simulink model "TRN_KAISIM"  (R2022a)
settings: Solver=FixedStepAuto  StartTime=0.0  StopTime=300  FixedStep=0.04  RelTol=1e-3
PreLoadFcn:
  | load('BusStructureTRNsensor.mat');
  | load('BusStructureTRN.mat');
InitFcn:
  | load('BusStructureTRNsensor.mat');
  | load('BusStructureTRN.mat');
undefined symbols (not defined in the file or in its folder): Altitude_INS, Latitude_INS, Longitude_INS, residual, Result_Prev, TimeTag_Prev, TRN, TRNlib
libraries: simulink_extras x18, sharedtransform x3
(part 1 of 4)
settings Model: Creator=HSU  LastModifiedBy=ASCL
settings OptimizationCC: DefaultParameterBehavior=Inlined  UseDivisionForNetSlopeComputation=on  GainParamInheritBuiltInType=on  UseFloatMulNetSlope=on  PassReuseOutputArgsAs=Individual arguments  ZeroExternalMemoryAtStartup=off  ZeroInternalMemoryAtStartup=off  LifeSpan=Inf  OptimizeBlockOrder=speed  DifferentSizesBufferReuse=on  EfficientTunableParamExpr=on
settings DebuggingCC: ParameterTunabilityLossMsg=error  UnconnectedInputMsg=warning  UnconnectedOutputMsg=warning  UnconnectedLineMsg=warning  SFUnexpectedBacktrackingDiag=warning  SFNoUnconditionalDefaultTransitionDiag=warning
settings HardwareCC: ProdBitPerPointer=32  ProdBitPerSizeT=32  ProdBitPerPtrDiffT=32  ProdLargestAtomicInteger=Long  ProdLargestAtomicFloat=Double  ProdEndianess=BigEndian  ProdWordSize=32  ProdLongLongMode=on  ProdHWDeviceType=Freescale->MPC83xx
settings ModelReferenceCC: ModelReferenceNumInstancesAllowed=Single
settings SFSimCC: SimCustomHeaderCode="#include \"MAP.h\""  SimUserSources=MAP.c  SimUserLibraries=WS2_32.LIB  MATLABDynamicMemAlloc=off
settings RTWCC: SystemTargetFile=ert.tlc  GenCodeOnly=on  TemplateMakefile=ert_default_tmf  GenerateReport=on  RTWUseSimCustomCode=on  CustomHeaderCode="#include \"MAP.h\""  CustomSource=MAP.c  CustomLibrary=WS2_32.LIB  BuildConfiguration=Faster Runs  LaunchReport=on  GenerateCodeMetricsReport=on  DLArmComputeVersion=19.05
settings CodeAppCC: ForceParamTrailComments=on  IgnoreCustomStorageClasses=off  OperatorAnnotations=on  SimulinkDataObjDesc=on  SFDataObjDesc=on  MATLABFcnDesc=on  InsertBlockDesc=on  StateflowObjectComments=on  MATLABSourceComments=on  EnableCustomComments=on  ReqsInCode=on
settings ERTTargetCC: TargetLangStandard=C99 (ISO)  UtilityFuncGeneration=Shared location  GenerateSampleERTMain=on  SuppressErrorStatus=on  SupportAbsoluteTime=off  SupportNonFinite=off  SupportComplex=off  SupportVariableSizeSignals=on  ParenthesesLevel=Standards  CastingMode=Standards  InlinedParameterPlacement=NonHierarchical  ERTCustomFileTemplate=example_file_process.tlc  PreserveIfCondition=on  ConvertIfToSwitch=off  EnableSignedLeftShifts=off  EnableSignedRightShifts=off

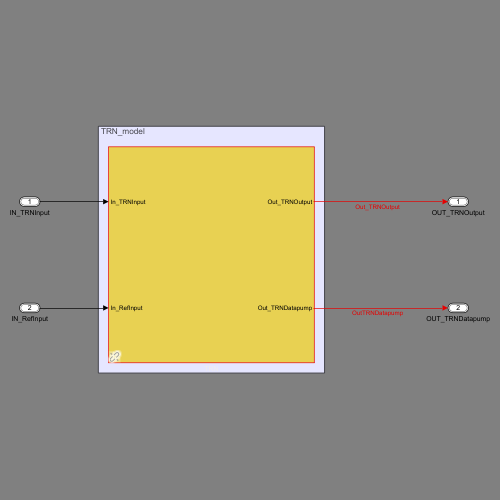
[thumbnail: Simulink's stored preview of the top-level diagram]
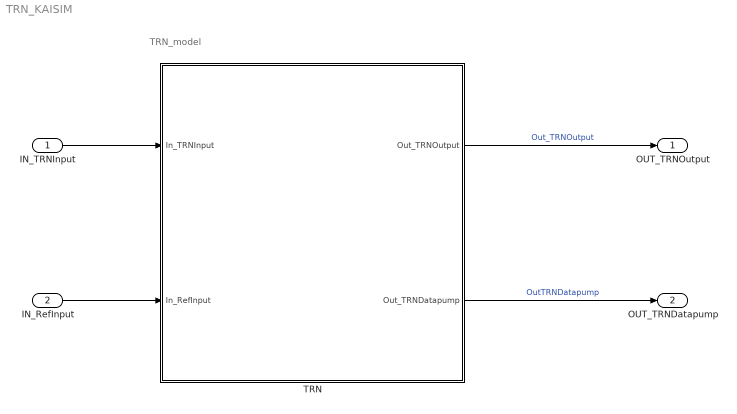
== system TRN_KAISIM ==
  note: TRN_model
  IN_TRNInput : Inport  OutDataTypeStr=Bus: TRNInput  Interpolate=off  BusOutputAsStruct=on
  IN_RefInput : Inport  Port=2  OutDataTypeStr=Bus: TRN_Ref  Interpolate=off  BusOutputAsStruct=on
  TRN : Subsystem  AncestorBlock=TRNlib/TRN
  OUT_TRNOutput : Outport  OutDataTypeStr=Bus: TRNOutput  BusOutputAsStruct=on
  OUT_TRNDatapump : Outport  Port=2  OutDataTypeStr=Bus: TRNDatapump  BusOutputAsStruct=on
  wires:
  IN_RefInput/1 -> TRN/2(In_RefInput)
  TRN/2(Out_TRNDatapump) -> OUT_TRNDatapump/1  "OutTRNDatapump"
  IN_TRNInput/1 -> TRN/1(In_TRNInput)
  TRN/1(Out_TRNOutput) -> OUT_TRNOutput/1  "Out_TRNOutput"

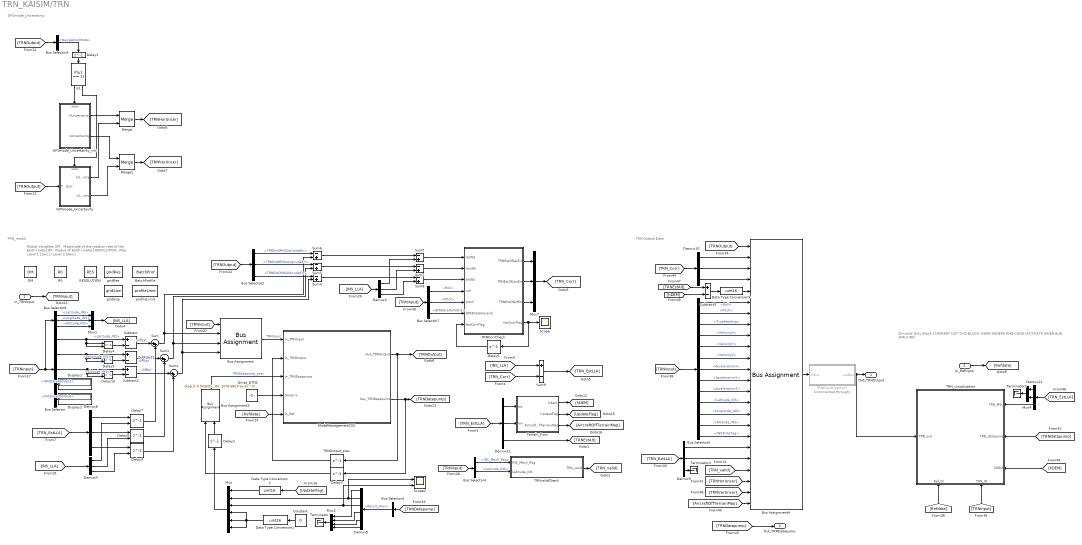
== system TRN_KAISIM/TRN ==
  note: GPSmode_Uncertainty
  note: Global Variables
      | OM : Magnitude of the rotation rate of the Earth [rad/s]
      | R0 : Radius of Earth [meter]
      | RESOLUTION : Map Level 1 [1arc] / Level 2 [3arc]
  note: TRN_modul
  note: TRN Output Data
  note: Simulink Only Block
      | COMMENT OUT THIS BLOCK WHEN GENERATING CODE
      | (ACTIVATE WHEN RUN SIMULINK)
  In_TRNInput : Inport  OutDataTypeStr=Bus: TRNInput
  In_RefInput : Inport  Port=2  OutDataTypeStr=Bus: TRN_Ref
  BatchProfile : DataStoreMemory  DataStoreName=BatchProf  ReadBeforeWriteMsg=warning  WriteAfterWriteMsg=warning  WriteAfterReadMsg=warning  ShowAdditionalParam=off  OutDataTypeStr=double  Dimensions=84200
  Bus Assignment : BusAssignment  AssignedSignals=Latitude_INS,Longitude_INS,Altitude_INS
  Bus Assignment3 : BusAssignment  AssignedSignals=Result_Prev
  Bus Assignment4 : BusAssignment  AssignedSignals=TRNEstOfINSLatitudeErr,TRNEstOfINSLongitudeErr,TRNEstOfINSAltitudeErr,TRNEstHeightAGL,TRN_Roll,TRN_Pitch,TRN_Yaw,TRN_VelocityX,TRN_VelocityY,TRN_VelocityZ,TRN_AccelerationX,TRN_AccelerationY,TRN_AccelerationZ,Latitude_INS,Longitude_INS,Altitude_INS,TRNTimeTag,TRNEstOfLatitude,TRNEstOfLongitude,TRN_valid,TRNHorUncertainty,TRNVerticalUncertainty,AircraftOffTerrainMap
  Bus Selector : BusSelector  OutputSignals=Latitude_INS,Longitude_INS,Altitude_INS,GPSDataNotValid,INSDataNotValid
  Bus Selector2 : BusSelector  OutputSignals=TRNEstOfINSLatitudeErr,TRNEstOfINSLongitudeErr,TRNEstOfINSAltitudeErr
  Bus Selector3 : BusSelector  OutputSignals=Result_Prev
  Bus Selector4 : BusSelector  OutputSignals=INS_Mech_flag,Latitude_INS
  Bus Selector5 : BusSelector  OutputSignals=Roll,Pitch,TrueHeading,VelocityX,VelocityY,VelocityZ,AccelerationX,AccelerationY,AccelerationZ,Latitude_INS,Longitude_INS,Altitude_INS,INSTimeTag
  Bus Selector6 : BusSelector  OutputSignals=Latitude_INS,Longitude_INS,Altitude_INS
  Bus Selector7 : BusSelector  OutputSignals=Roll,Pitch,GPSDataNotValid
  Bus Selector9 : BusSelector  OutputSignals=NavigationMode
  Constant : Constant  Value=0
  Data Type Conversion1 : DataTypeConversion  OutDataTypeStr=uint16  SaturateOnIntegerOverflow=off  RndMeth=Floor
  Data Type Conversion2 : DataTypeConversion  OutDataTypeStr=uint16  SaturateOnIntegerOverflow=off  RndMeth=Floor
  Data Type Conversion3 : DataTypeConversion  OutDataTypeStr=uint16  RndMeth=Nearest  SaturateOnIntegerOverflow=off
  Delay1 : Delay  DelayLength=1  InitialCondition=1
  Delay10 : Delay  DelayLength=1  InitialConditionSource=Input port  InitialCondition=35.2*pi/180
      settings: InputPortMap=u0,p4
  Delay2 : Delay  DelayLength=1  InitialCondition=0
  Delay3 : Delay  DelayLength=1  InitialCondition=0
  Delay4 : Delay  DelayLength=1  InitialConditionSource=Input port  InitialCondition=35.2*pi/180
      settings: InputPortMap=u0,p4
  Delay5 : Delay  DelayLength=1  InitialConditionSource=Input port  InitialCondition=35.2*pi/180
      settings: InputPortMap=u0,p4
  Delay6 : Delay  DelayLength=1
  Delay7 : Delay  DelayLength=1  InitialConditionSource=Input port  InitialCondition=0
      settings: InputPortMap=u0,p4
  Delay8 : Delay  DelayLength=1  InitialConditionSource=Input port  InitialCondition=0
      settings: InputPortMap=u0,p4
  Delay9 : Delay  DelayLength=1  InitialConditionSource=Input port  InitialCondition=0
      settings: InputPortMap=u0,p4
  Demux{3..4,8..12} (7 alike) : Demux  Outputs=3
  Demux5 : Demux  Outputs=6
  Display1 : Display
  Display2 : Display
  GPSmode_Uncertainty : Subsystem  TreatAsAtomicUnit=on
  GPSmode_Uncertainty_init : Subsystem  TreatAsAtomicUnit=on
  If1 : If  IfExpression=u1 == 1
  Merge : Merge
  Merge1 : Merge
  ModeManagementCSU : Stateflow chart  TreatAsAtomicUnit=on
      settings: RTWSystemCode=Nonreusable function  RTWFcnNameOpts=Use subsystem name
  Mux : Mux  Inputs=6
  Mux1 : Mux  Inputs=3
  Mux2 : Mux
  Mux4 : Mux  Inputs=2
  Mux7 : Mux  Inputs=3
  OM : DataStoreMemory  DataStoreName=OM  ReadBeforeWriteMsg=warning  WriteAfterWriteMsg=warning  WriteAfterReadMsg=warning  InitialValue=7.27e-5  ShowAdditionalParam=off
  Qmat_DTNS : Constant  Value=diag(([-0.043633231299858 0.06302577854424 -0.431484176187487 784 -1078 686]*1e-6).^2)
  R0 : DataStoreMemory  DataStoreName=R0  ReadBeforeWriteMsg=warning  WriteAfterWriteMsg=warning  WriteAfterReadMsg=warning  InitialValue=6378000  ShowAdditionalParam=off
  RESOLUTION : DataStoreMemory  DataStoreName=RES  ReadBeforeWriteMsg=warning  WriteAfterWriteMsg=warning  WriteAfterReadMsg=warning  InitialValue=1 * 0.000277777777777777 * 0.0174532925199433  ShowAdditionalParam=off  OutDataTypeStr=double
  Scope : Scope
  Scope2 : Scope  NumInputPorts=2
  Subtract{,1..3} (4 alike) : Sum  Inputs=+-
  Sum : Sum  Inputs=|++
  Sum1 : Sum  Inputs=|++
  Sum2 : Sum  Inputs=|++
  Sum{3..8} (6 alike) : Sum  Inputs=-+
  Sum9 : Sum  Inputs=+-
  TRNCorrCheck : MATLAB Function  TreatAsAtomicUnit=on
      settings: RTWSystemCode=Nonreusable function  RTWFcnNameOpts=Use subsystem name
  TRNEventInjector1 : MATLAB Function  Commented=through  TreatAsAtomicUnit=on
  TRNOutput_prev : Delay  DelayLength=1  InitialCondition=struct('NavigationMode', false);
  TRN_visualization : Subsystem
      settings: PortSchema="{\"entries\":[{\"content\":{\"sides\":[{\"content\":{\"connectorIds\":[\"In1\",\"In2\",\"In3\"]},\"type\":\"ConnectorPlacement.EquallySpacedRectSide\",\"uuid\":\"9b00cbc4-ca0d-429d-9536-38963fe71bc1\"},{\"content\":{\"connectorIds\":[\"In6\"],\"side\":\"RIGHT\"},\"type\":\"ConnectorPlacement.EquallySpacedRectSide\",\"uuid\":\"1db309fb-4b82-499a-a8dc-4a1ba85275fb\"},{\"content\":{\"connectorIds\":[\"In4\",\"In5\"],\"side\":\"TOP\"},\"type\":\"ConnectorPlacement.EquallySpacedRectSide\",\"uuid\":\"7e2d2316-30f0-423f-b46b-636ee0f4a770\"}]},\"type\":\"ConnectorPlacement.EquallySpacedConnector\",\"uuid\":\"aa6e905d-ed4c-45ad-a850-3c33939aad22\"}],\"packageUris\":[\"http://schema.mathworks.com/mf0/Connector/R2020b\"],\"version\":\"1.0\"}"
  TRNvalidCheck : MATLAB Function  TreatAsAtomicUnit=on
      settings: RTWSystemCode=Nonreusable function  RTWFcnNameOpts=Use subsystem name
  Terminator : Terminator
  Terminator3 : Terminator
  Terminator4 : Terminator
  Terrain_Func : Subsystem
  gridRes : DataStoreMemory  DataStoreName=gridRes  ReadBeforeWriteMsg=warning  WriteAfterWriteMsg=warning  WriteAfterReadMsg=warning  InitialValue=0.3  ShowAdditionalParam=off  OutDataTypeStr=double
  gridSize : DataStoreMemory  DataStoreName=gridSize  ReadBeforeWriteMsg=warning  WriteAfterWriteMsg=warning  WriteAfterReadMsg=warning  InitialValue=20  ShowAdditionalParam=off  OutDataTypeStr=double
  profileLimit : DataStoreMemory  DataStoreName=profileLimit  ReadBeforeWriteMsg=warning  WriteAfterWriteMsg=warning  WriteAfterReadMsg=warning  InitialValue=20  ShowAdditionalParam=off  OutDataTypeStr=uint16
  Out_TRNOutput : Outport  OutDataTypeStr=Bus: TRNOutput  VectorParamsAs1DForOutWhenUnconnected=off
  Out_TRNDatapump : Outport  Port=2  OutDataTypeStr=Bus: TRNDatapump  VectorParamsAs1DForOutWhenUnconnected=off
  wires:
  If1/1 -> GPSmode_Uncertainty_init/Action
  If1/2 -> GPSmode_Uncertainty/Action
  GPSmode_Uncertainty_init/1(hUncertainty) -> Merge/1
  GPSmode_Uncertainty/1(hUncertainty) -> Merge/2
  GPSmode_Uncertainty_init/2(vUncertainty) -> Merge1/1
  GPSmode_Uncertainty/2(vUncertainty) -> Merge1/2
  Bus Selector9/1 -> Delay1/1  "<NavigationMode>"
  Merge/1 -> [TRNHorUncer]
  Merge1/1 -> [TRNVerUncer]
  [TRNOutput] -> Bus Selector9/1
  [TRNOutput] -> GPSmode_Uncertainty/1(TRNOutput)
  Delay1/1 -> If1/1
  Delay10/1 -> Subtract2/2
  [TRN_Corr] -> Sum9/2
  Mux/1 -> Delay2/1
  TRNCorrCheck/4(NotCorrFlag) -> Scope/1, Delay6/1
  Bus Selector/5 -> Display2/1  "<INSDataNotValid>"
  In_TRNInput/1 -> [TRNinput]
  Bus Selector/4 -> Display1/1  "<GPSDataNotValid>"
  Bus Selector6/1 -> Mux1/1  "<Latitude_INS>"
  [TRNOutput] -> Bus Selector2/1
  Bus Assignment3/1 -> ModeManagementCSU/3(In_TRNDatapump)  "TRNDatapump_prev"
  [INS_LLA] -> Demux4/1
  Demux4/3 -> Delay9/2
  Delay7/1 -> Sum/2
  Bus Selector7/3 -> TRNCorrCheck/6(GPSDataNotvalid)  "<GPSDataNotValid>"
  Demux4/2 -> Delay8/2
  Demux4/1 -> Delay7/2
  [TRNinput] -> Bus Selector7/1
  ModeManagementCSU/2(Out_TRNDatapump) -> Delay3/1, [TRNDatapump]
  Bus Selector7/1 -> TRNCorrCheck/4(roll)  "<Roll>"
  [TRNinput] -> Bus Selector6/1, Bus Selector/1
  [INS_LLA] -> Demux3/1
  Bus Selector6/2 -> Mux1/2  "<Longitude_INS>"
  Demux11/1 -> Terrain_Func/1(lat)
  Delay6/1 -> TRNCorrCheck/7("NotCorrFlag ")
  Sum9/1 -> [TRN_EstLLA]
  Bus Selector6/3 -> Mux1/3  "<Altitude_INS>"
  Mux7/1 -> [TRN_Corr]
  TRNCorrCheck/1(TRNEstOfLatErr) -> Mux7/1
  Subtract2/1 -> Sum2/1  "diffAlt"
  Delay9/1 -> Sum2/2
  [TRN_EstLLA] -> Demux8/1
  Demux8/3 -> Delay9/1
  Sum8/1 -> TRNCorrCheck/3(altINS)
  Sum7/1 -> TRNCorrCheck/2(lonINS)
  Sum/1 -> Sum6/2, Bus Assignment/2
  Bus Selector2/1 -> Sum6/1  "<TRNEstOfINSLatitudeErr>"
  Subtract/1 -> Sum/1  "diffLat"
  Delay8/1 -> Sum1/2
  Sum3/1 -> Sum7/1
  TRNOutput_prev/1 -> ModeManagementCSU/2(In_TRNOutput)
  Bus Selector/2 -> Subtract1/1, Delay5/2, Delay5/1  "<Longitude_INS>"
  Delay5/1 -> Subtract1/2
  Subtract1/1 -> Sum1/1  "diffLon"
  Bus Assignment/1 -> ModeManagementCSU/1(In_TRNInput)  "TRNInput"
  [INS_LLA] -> Sum9/1
  [TRNinput] -> Bus Assignment/1
  Terrain_Func/1(hdem) -> [hDEM]
  Delay4/1 -> Subtract/2
  Sum5/1 -> TRNCorrCheck/1(latINS)
  Demux3/1 -> Sum5/2
  Demux11/2 -> Terrain_Func/2(lon)
  Bus Selector2/2 -> Sum3/1  "<TRNEstOfINSLongitudeErr>"
  Demux3/3 -> Sum8/2
  Mux1/1 -> [INS_LLA]
  Demux3/2 -> Sum7/2
  Demux8/1 -> Delay7/1
  [TRN_EstLLA] -> Demux11/1
  [UpdateFlag] -> Data Type Conversion2/1
  Sum1/1 -> Sum3/2, Bus Assignment/3
  Terrain_Func/3(AircraftOffTerrainMap) -> [AircraftOffTerrainMap]
  Delay3/1 -> Bus Assignment3/1
  Demux11/3 -> [TRNEstAlt]
  Terrain_Func/2(Updateflag) -> [UpdateFlag]
  Constant/1 -> Data Type Conversion1/1
  TRNvalidCheck/1(TRN_valid) -> [TRN_valid]
  TRNCorrCheck/2(TRNEstOfLonErr) -> Mux7/2
  Demux8/2 -> Delay8/1
  Bus Selector/1 -> Delay4/2, Delay4/1, Subtract/1  "<Latitude_INS>"
  Bus Selector/3 -> Delay10/1, Delay10/2, Subtract2/1  "<Altitude_INS>"
  Delay2/1 -> Bus Assignment3/2
  TRNCorrCheck/3(TRNEstOfaltErr) -> Mux7/3
  Bus Selector2/3 -> Sum4/1  "<TRNEstOfINSAltitudeErr>"
  Bus Selector7/2 -> TRNCorrCheck/5(pitch)  "<Pitch>"
  ModeManagementCSU/1(Out_TRNOutput) -> [TRNOutput], TRNOutput_prev/1
  [TRNinput] -> Bus Selector4/1
  Data Type Conversion1/1 -> Mux/4, Mux/6, Mux/5
  Data Type Conversion2/1 -> Mux/1
  Sum2/1 -> Sum4/2, Bus Assignment/4
  Bus Selector4/1 -> TRNvalidCheck/1(INS_Mech_flag)  "<INS_Mech_flag>"
  Bus Selector4/2 -> TRNvalidCheck/2(Latitude_INS)  "<Latitude_INS>"
  Qmat_DTNS/1 -> ModeManagementCSU/4(Qmatrix)
  [Refdata] -> ModeManagementCSU/5(In_Ref)
  Bus Selector3/1 -> Demux5/1  "<Result_Prev>"
  [TRNDatapump] -> Bus Selector3/1
  Sum4/1 -> Sum8/1
  Sum6/1 -> Sum5/1
  Demux5/2 -> Mux/2, Scope2/1
  Demux5/3 -> Mux/3, Scope2/2
  Mux2/1 -> Terminator/1
  Demux5/1 -> Mux2/1
  Demux5/4 -> Mux2/2
  Demux5/5 -> Mux2/3
  Demux5/6 -> Mux2/4
  [TRNDatapump] -> Out_TRNDatapump/1
  Bus Selector5/8 -> Bus Assignment4/13  "<AccelerationY>"
  [TRNDatapump] -> TRN_visualization/2(TRN_datapump)
  Demux9/3 -> Terminator4/1
  [Refdata] -> TRN_visualization/5(Ref_IN)
  Bus Selector5/12 -> Bus Assignment4/17  "<Altitude_INS>"
  [TRN_EstLLA] -> Demux12/1
  Bus Selector5/3 -> Bus Assignment4/8  "<TrueHeading>"
  Demux9/2 -> Bus Assignment4/20
  [TRNVerUncer] -> Bus Assignment4/23
  [hDEM] -> Subtract3/2
  Bus Selector5/6 -> Bus Assignment4/11  "<VelocityZ>"
  [TRNOutput] -> Bus Assignment4/1
  Demux12/1 -> Mux4/1
  [TRN_EstLLA] -> Demux9/1
  Bus Selector5/2 -> Bus Assignment4/7  "<Pitch>"
  [hDEM] -> TRN_visualization/1(hDEM)
  [AircraftOffTerrainMap] -> Bus Assignment4/24
  Demux12/3 -> TRN_visualization/3(TRN_MSL)
  [TRN_Corr] -> Demux10/1
  Demux10/1 -> Bus Assignment4/2
  [TRNinput] -> TRN_visualization/4(TRN_IN)
  Bus Assignment4/1 -> TRNEventInjector1/1(inBus)
  Bus Selector5/1 -> Bus Assignment4/6  "<Roll>"
  Bus Selector5/4 -> Bus Assignment4/9  "<VelocityX>"
  Bus Selector5/13 -> Bus Assignment4/18  "<INSTimeTag>"
  Bus Selector5/5 -> Bus Assignment4/10  "<VelocityY>"
  Demux10/2 -> Bus Assignment4/3
  Bus Selector5/10 -> Bus Assignment4/15  "<Latitude_INS>"
  Data Type Conversion3/1 -> Bus Assignment4/5
  Bus Selector5/7 -> Bus Assignment4/12  "<AccelerationX>"
  In_RefInput/1 -> [Refdata]
  Demux9/1 -> Bus Assignment4/19
  Mux4/1 -> Terminator3/1
  Demux12/2 -> Mux4/2
  Bus Selector5/9 -> Bus Assignment4/14  "<AccelerationZ>"
  Demux10/3 -> Bus Assignment4/4
  Subtract3/1 -> Data Type Conversion3/1
  [TRNinput] -> Bus Selector5/1
  [TRN_valid] -> Bus Assignment4/21
  Bus Selector5/11 -> Bus Assignment4/16  "<Longitude_INS>"
  [TRNHorUncer] -> Bus Assignment4/22
  [TRNEstAlt] -> Subtract3/1
  TRNEventInjector1/1(outBus) -> TRN_visualization/6(TRN_out), Out_TRNOutput/1

== system TRN_KAISIM/TRN/GPSmode_Uncertainty ==
  TRNOutput : Inport
  Action Port : ActionPort  ActionPortLabel=else
  Bus Selector : BusSelector  OutputSignals=TRNHorUncertainty,TRNVerticalUncertainty
  Scope : Scope  NumInputPorts=2
  hUncertainty : Outport
  vUncertainty : Outport  Port=2
  wires:
  TRNOutput/1 -> Bus Selector/1
  Bus Selector/1 -> Scope/1, hUncertainty/1  "<TRNHorUncertainty>"
  Bus Selector/2 -> vUncertainty/1, Scope/2  "<TRNVerticalUncertainty>"

== system TRN_KAISIM/TRN/GPSmode_Uncertainty_init ==
  Action Port : ActionPort  ActionPortLabel=if(u1 == 1)
  Uncertainty_init : MATLAB Function  TreatAsAtomicUnit=on
  hUncertainty : Outport
  vUncertainty : Outport  Port=2
  wires:
  Uncertainty_init/1(hUncertainty) -> hUncertainty/1
  Uncertainty_init/2(vUncertainty) -> vUncertainty/1

== system TRN_KAISIM/TRN/ModeManagementCSU/AcquisitionCSU ==
  In_TRNInput : Inport  OutDataTypeStr=Bus: TRNInput  PortDimensions=1
  In_TRNDatapump : Inport  Port=2  OutDataTypeStr=Bus: TRNDatapump  PortDimensions=1
  f : TriggerPort  TriggerType=function-call  VariantControl=Variant
      settings: CopyFcn=Stateflow.SLINSF.SimulinkMan.removeBlockPreDeleteFcn  PreDeleteFcn=Stateflow.SLINSF.SimulinkMan.unsafePredeleteFcn
  AcquisitionCSU : Subsystem  TreatAsAtomicUnit=on
      settings: RTWSystemCode=Nonreusable function  RTWFcnNameOpts=Use subsystem name
  MAD : Outport  VectorParamsAs1DForOutWhenUnconnected=off
  profileCnt : Outport  Port=2  VectorParamsAs1DForOutWhenUnconnected=off
  posUpdate : Outport  Port=3  VectorParamsAs1DForOutWhenUnconnected=off
  residual : Outport  Port=4  VectorParamsAs1DForOutWhenUnconnected=off
  wires:
  In_TRNInput/1 -> AcquisitionCSU/1(In_TRNInput)
  In_TRNDatapump/1 -> AcquisitionCSU/2(In_TRNDatapump)
  AcquisitionCSU/1(MAD) -> MAD/1
  AcquisitionCSU/2(profileCnt) -> profileCnt/1
  AcquisitionCSU/3(posUpdate) -> posUpdate/1
  AcquisitionCSU/4(residual) -> residual/1

== system TRN_KAISIM/TRN/ModeManagementCSU/CorrelationValid ==
  In_TRNDatapump : Inport  OutDataTypeStr=Bus: TRNDatapump  PortDimensions=1
  In_TRNInput : Inport  Port=2  OutDataTypeStr=Bus: TRNInput  PortDimensions=1
  posUpdate : Inport  Port=3  OutDataTypeStr=double  PortDimensions=2
  In_Ref : Inport  Port=4  OutDataTypeStr=Bus: TRN_Ref  PortDimensions=1
  f : TriggerPort  TriggerType=function-call  VariantControl=Variant
      settings: CopyFcn=Stateflow.SLINSF.SimulinkMan.removeBlockPreDeleteFcn  PreDeleteFcn=Stateflow.SLINSF.SimulinkMan.unsafePredeleteFcn
  Bus Selector1 : BusSelector  OutputSignals=MAD,profileCnt
  Bus Selector2 : BusSelector  OutputSignals=GPSDataNotValid
  Bus Selector3 : BusSelector  OutputSignals=Latitude,Longitude
  CorrelationValid function : MATLAB Function  TreatAsAtomicUnit=on
  Terminator1 : Terminator
  Terminator4 : Terminator
  TRNEstLatErr : Outport  VectorParamsAs1DForOutWhenUnconnected=off
  TRNEstLonErr : Outport  Port=2  VectorParamsAs1DForOutWhenUnconnected=off
  TRNEstAltErr : Outport  Port=3
  profileCnt : Outport  Port=4  OutDataTypeStr=uint32
  NavigationMode : Outport  Port=5  OutDataTypeStr=boolean
  AircraftPositionCorrectionValid : Outport  Port=6
  wires:
  In_TRNDatapump/1 -> Bus Selector1/1
  Bus Selector1/2 -> CorrelationValid function/3("profileCnt ")  "<profileCnt>"
  Bus Selector2/1 -> CorrelationValid function/4(GPSDataNotValid)  "<GPSDataNotValid>"
  In_TRNInput/1 -> Bus Selector2/1
  Bus Selector1/1 -> CorrelationValid function/2(MAD)  "<MAD>"
  CorrelationValid function/1(TRNEstOfINSLatitudeErr) -> TRNEstLatErr/1
  CorrelationValid function/2(TRNEstOfINSLongitudeErr) -> TRNEstLonErr/1
  CorrelationValid function/3(TRNEstOfINSAltitudeErr) -> TRNEstAltErr/1
  CorrelationValid function/4(profileCnt) -> profileCnt/1
  CorrelationValid function/5(NavigationMode) -> NavigationMode/1
  CorrelationValid function/6(AircraftPositionCorrectionValid) -> AircraftPositionCorrectionValid/1
  posUpdate/1 -> CorrelationValid function/1(posUpdate)
  In_Ref/1 -> Bus Selector3/1
  Bus Selector3/1 -> Terminator4/1  "<Latitude>"
  Bus Selector3/2 -> Terminator1/1  "<Longitude>"

== system TRN_KAISIM/TRN/ModeManagementCSU/TrackingCSU ==
  In_TRNInput : Inport  OutDataTypeStr=Bus: TRNInput  PortDimensions=1
  Qmatrix : Inport  Port=2  OutDataTypeStr=double  PortDimensions=[6 6]
  In_TRNDatapump : Inport  Port=3  OutDataTypeStr=Bus: TRNDatapump  PortDimensions=1
  f : TriggerPort  TriggerType=function-call  VariantControl=Variant
      settings: CopyFcn=Stateflow.SLINSF.SimulinkMan.removeBlockPreDeleteFcn  PreDeleteFcn=Stateflow.SLINSF.SimulinkMan.unsafePredeleteFcn
  TrackingCSU_20230430 : Subsystem  TreatAsAtomicUnit=on
      settings: RTWSystemCode=Nonreusable function  RTWFcnNameOpts=Use subsystem name
  latINSErrTRN : Outport  VectorParamsAs1DForOutWhenUnconnected=off
  lonINSErrTRN : Outport  Port=2  VectorParamsAs1DForOutWhenUnconnected=off
  altINSErrTRN : Outport  Port=3  VectorParamsAs1DForOutWhenUnconnected=off
  hUncertainty : Outport  Port=4  VectorParamsAs1DForOutWhenUnconnected=off
  vUncertainty : Outport  Port=5  VectorParamsAs1DForOutWhenUnconnected=off
  Out_TRNDatapump : Outport  Port=6  VectorParamsAs1DForOutWhenUnconnected=off
  wires:
  In_TRNInput/1 -> [In_TRNinput]
  Qmatrix/1 -> [Qmat]
  In_TRNDatapump/1 -> [In_TRNDatapump]
  [In_TRNinput] -> TrackingCSU_20230430/1(In_TRNInput)
  [In_TRNDatapump] -> TrackingCSU_20230430/3(In_TRNDatapump)
  TrackingCSU_20230430/1(latINSErrTRN) -> latINSErrTRN/1
  TrackingCSU_20230430/2(lonINSErrTRN) -> lonINSErrTRN/1
  TrackingCSU_20230430/3(altINSErrTRN) -> altINSErrTRN/1
  TrackingCSU_20230430/5(vUncertainty) -> vUncertainty/1
  [Qmat] -> TrackingCSU_20230430/2(Qmatrix)
  TrackingCSU_20230430/4(hUncertainty) -> hUncertainty/1
  TrackingCSU_20230430/6(TRN_Datapump) -> Out_TRNDatapump/1

== system TRN_KAISIM/TRN/ModeManagementCSU/ValidityCheck ==
  continuousValid : Inport  OutDataTypeStr=boolean  PortDimensions=1
  latINSErrTRN : Inport  Port=2  OutDataTypeStr=double  PortDimensions=1
  lonINSErrTRN : Inport  Port=3  OutDataTypeStr=double  PortDimensions=1
  altINSErrTRN : Inport  Port=4  OutDataTypeStr=double  PortDimensions=1
  Result_prev : Inport  Port=5  OutDataTypeStr=uint16  PortDimensions=6
  f : TriggerPort  TriggerType=function-call  VariantControl=Variant
      settings: CopyFcn=Stateflow.SLINSF.SimulinkMan.removeBlockPreDeleteFcn  PreDeleteFcn=Stateflow.SLINSF.SimulinkMan.unsafePredeleteFcn
  Data Type Conversion : DataTypeConversion  OutDataTypeStr=boolean  SaturateOnIntegerOverflow=off  RndMeth=Floor
  Demux : Demux  Outputs=6
  Mux : Mux  Inputs=5
  Terminator : Terminator
  ValidityCheck : MATLAB Function  TreatAsAtomicUnit=on
      settings: RTWFcnNameOpts=Use subsystem name
  TRNEstOfINSLatitudeErr : Outport  VectorParamsAs1DForOutWhenUnconnected=off
  TRNEstOfINSLongitudeErr : Outport  Port=2
  TRNEstOfINSAltitudeErr : Outport  Port=3
  AircraftPositionCorrectionValid : Outport  Port=4  OutDataTypeStr=boolean
  wires:
  ValidityCheck/4(AircraftPositionCorrectionValid) -> AircraftPositionCorrectionValid/1
  continuousValid/1 -> ValidityCheck/1(continuousValid)
  latINSErrTRN/1 -> ValidityCheck/2(latINSErrTRN)
  lonINSErrTRN/1 -> ValidityCheck/3(lonINSErrTRN)
  altINSErrTRN/1 -> ValidityCheck/4(altINSErrTRN)
  ValidityCheck/3(TRNEstOfINSAltitudeErr) -> TRNEstOfINSAltitudeErr/1
  ValidityCheck/2(TRNEstOfINSLongitudeErr) -> TRNEstOfINSLongitudeErr/1
  ValidityCheck/1(TRNEstOfINSLatitudeErr) -> TRNEstOfINSLatitudeErr/1
  Result_prev/1 -> Demux/1
  Data Type Conversion/1 -> ValidityCheck/5(velFlag)
  Demux/3 -> Data Type Conversion/1
  Demux/1 -> Mux/1
  Demux/2 -> Mux/2
  Demux/4 -> Mux/3
  Demux/5 -> Mux/4
  Demux/6 -> Mux/5
  Mux/1 -> Terminator/1

== system TRN_KAISIM/TRN/ModeManagementCSU/Ver_FlightPath_Angle ==
  In_TRNInput : Inport  OutDataTypeStr=Bus: TRNInput  PortDimensions=1
  f : TriggerPort  TriggerType=function-call  VariantControl=Variant
      settings: CopyFcn=Stateflow.SLINSF.SimulinkMan.removeBlockPreDeleteFcn  PreDeleteFcn=Stateflow.SLINSF.SimulinkMan.unsafePredeleteFcn
  Bus Selector1 : BusSelector  OutputSignals=VelocityX,VelocityY,VelocityZ,Roll,Pitch,TrueHeading
  Degrees to Radians1 : simulink_extras/Transformations/Degrees to Radians
  Degrees to Radians2 : simulink_extras/Transformations/Degrees to Radians
  Degrees to Radians3 : simulink_extras/Transformations/Degrees to Radians
  FlightPath_Angle : MATLAB Function  TreatAsAtomicUnit=on
  Matrix Multiply1 : Product  Multiplication=Matrix(*)
  Mux : Mux  Inputs=3
  Mux2 : Mux  Inputs=3
  Rotation Angles to Direction Cosine Matrix : sharedtransform/Rotation Angles to Direction Cosine Matrix  rotationOrder=ZYX  aMode=aMode
      settings: SourceProductBaseCode=AE,PW,DR,MT,VE
  Selector : Selector  InputPortWidth=3  IndexOptions=Index vector (dialog)  Indices=[3 2 1]  OutputSizes=1
  Transpose : Math  Operator=transpose  SignedPower=on
  TRN_Ver_FlightPath_Angle : Outport  OutDataTypeStr=double
  wires:
  Bus Selector1/4 -> Degrees to Radians1/1  "<Roll>"
  Transpose/1 -> Matrix Multiply1/1
  Selector/1 -> Rotation Angles to Direction Cosine Matrix/1
  FlightPath_Angle/1(TRN_Ver_FlightPath_Angle) -> TRN_Ver_FlightPath_Angle/1
  Degrees to Radians1/1 -> Mux/1
  Bus Selector1/1 -> Mux2/1  "<VelocityX>"
  In_TRNInput/1 -> Bus Selector1/1
  Bus Selector1/6 -> Degrees to Radians3/1  "<TrueHeading>"
  Mux2/1 -> Matrix Multiply1/2
  Degrees to Radians3/1 -> Mux/3
  Degrees to Radians2/1 -> Mux/2
  Bus Selector1/5 -> Degrees to Radians2/1  "<Pitch>"
  Bus Selector1/3 -> Mux2/3  "<VelocityZ>"
  Mux/1 -> Selector/1
  Matrix Multiply1/1 -> FlightPath_Angle/1(vNED)
  Rotation Angles to Direction Cosine Matrix/1 -> Transpose/1
  Bus Selector1/2 -> Mux2/2  "<VelocityY>"

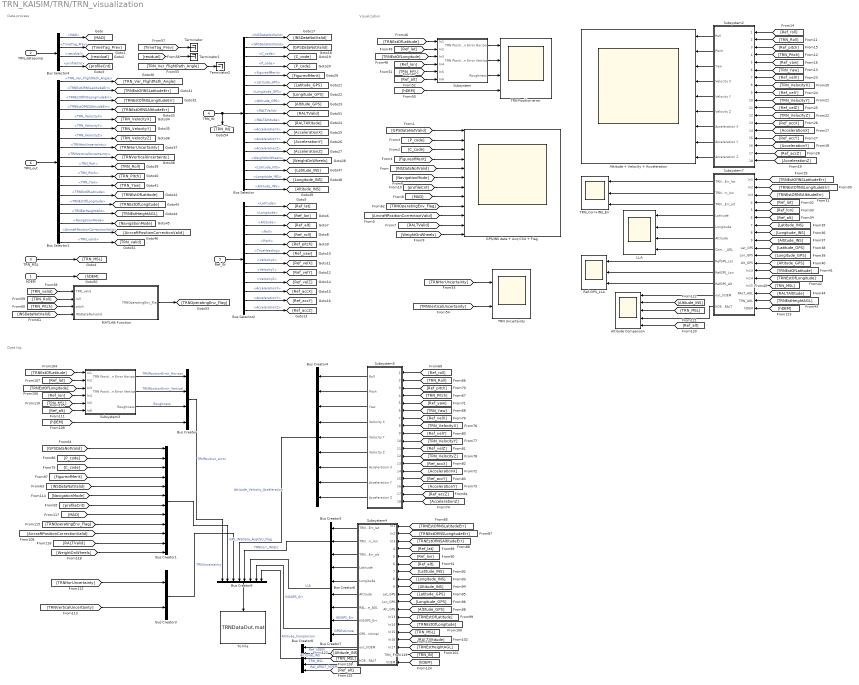
== system TRN_KAISIM/TRN/TRN_visualization ==
  note: Visualization
  note: Data process
  note: Data log
  hDEM : Inport
  TRN_datapump : Inport  Port=2
  TRN_MSL : Inport  Port=3
  TRN_IN : Inport  Port=4
  Ref_IN : Inport  Port=5
  TRN_out : Inport  Port=6
  Altitude Comparison : Scope  NumInputPorts=5
  Attitude + Velocity + Acceleration : Scope  NumInputPorts=9
  Bus Creator : BusCreator  Inputs=4
  Bus Creator1 : BusCreator  Inputs=12
  Bus Creator3 : BusCreator  Inputs=2
  Bus Creator4 : BusCreator  Inputs=9
  Bus Creator5 : BusCreator  Inputs=3
  Bus Creator6 : BusCreator  Inputs=4
  Bus Creator7 : BusCreator  Inputs=2
  Bus Creator8 : BusCreator  Inputs=5
  Bus Creator9 : BusCreator  Inputs=8
  Bus Selector : BusSelector  OutputSignals=INSDataNotValid,GPSDataNotValid,C_code,P_code,FigureofMerit,Latitude_GPS,Longitude_GPS,Altitude_GPS,RALTValid,RALTAltitude,AccelerationX,AccelerationY,AccelerationZ,WeightOnWheels,Latitude_INS,Longitude_INS,Altitude_INS
  Bus Selector1 : BusSelector  OutputSignals=TRN_Ver_FlightPath_Angle,TRNEstOfINSLatitudeErr,TRNEstOfINSLongitudeErr,TRNEstOfINSAltitudeErr,TRN_VelocityX,TRN_VelocityY,TRN_VelocityZ,TRNHorUncertainty,TRNVerticalUncertainty,TRN_Roll,TRN_Pitch,TRN_Yaw,TRNEstOfLatitude,TRNEstOfLongitude,TRNEstHeightAGL,NavigationMode,AircraftPositionCorrectionValid,TRN_valid
  Bus Selector2 : BusSelector  OutputSignals=Latitude,Longitude,Altitude,Roll,Pitch,TrueHeading,VelocityX,VelocityY,VelocityZ,AccelerationX,AccelerationY,AccelerationZ
  Bus Selector4 : BusSelector  OutputSignals=MAD,TimeTag_Prev,residual,profileCnt
  GPS/INS data + Acq CSU + Flag : Scope  NumInputPorts=12
  LLA : Scope  NumInputPorts=4
  MATLAB Function : MATLAB Function  TreatAsAtomicUnit=on
  Ref-GPS_LLA : Scope  NumInputPorts=3
  Subsystem : Subsystem
  Subsystem2 : Subsystem
  Subsystem3 : Subsystem
  Subsystem4 : Subsystem
  Subsystem5 : Subsystem
  Subsystem7 : Subsystem
  TRN Position error : Scope  NumInputPorts=4
  TRN Uncertainty : Scope  NumInputPorts=2
  TRN_Corr+INS_Err : Scope  NumInputPorts=3
  Terminator : Terminator
  Terminator1 : Terminator
  Terminator2 : Terminator
  To File : ToFile  Filename=TRNDataOut.mat  MatrixName=Out_TRNData  SaveFormat=Timeseries
  wires:
  TRN_IN/1 -> Bus Selector/1, [TRN_IN]
  Ref_IN/1 -> Bus Selector2/1
  TRN_out/1 -> Bus Selector1/1
  TRN_datapump/1 -> Bus Selector4/1
  Bus Selector4/1 -> [MAD]  "<MAD>"
  Bus Selector4/2 -> [TimeTag_Prev]  "<TimeTag_Prev>"
  Bus Selector4/3 -> [residual]  "<residual>"
  Bus Selector4/4 -> [profileCnt]  "<profileCnt>"
  TRN_MSL/1 -> [TRN_MSL]
  Bus Selector2/1 -> [Ref_lat]  "<Latitude>"
  Bus Selector2/2 -> [Ref_lon]  "<Longitude>"
  Bus Selector2/12 -> [Ref_accZ]  "<AccelerationZ>"
  Bus Selector2/3 -> [Ref_alt]  "<Altitude>"
  Bus Selector2/4 -> [Ref_roll]  "<Roll>"
  Bus Selector2/5 -> [Ref_pitch]  "<Pitch>"
  Bus Selector2/6 -> [Ref_yaw]  "<TrueHeading>"
  Bus Selector2/7 -> [Ref_velX]  "<VelocityX>"
  Bus Selector2/8 -> [Ref_velY]  "<VelocityY>"
  Bus Selector2/9 -> [Ref_velZ]  "<VelocityZ>"
  Bus Selector2/10 -> [Ref_accX]  "<AccelerationX>"
  Bus Selector2/11 -> [Ref_accY]  "<AccelerationY>"
  Bus Selector/2 -> [GPSDataNotValid]  "<GPSDataNotValid>"
  Bus Selector/3 -> [C_code]  "<C_code>"
  Bus Selector/4 -> [P_code]  "<P_code>"
  Bus Selector/6 -> [Latitude_GPS]  "<Latitude_GPS>"
  Bus Selector/7 -> [Longitude_GPS]  "<Longitude_GPS>"
  Bus Selector/8 -> [Altitude_GPS]  "<Altitude_GPS>"
  Bus Selector/10 -> [RALTAltitude]  "<RALTAltitude>"
  Bus Selector/11 -> [AccelerationX]  "<AccelerationX>"
  Bus Selector/12 -> [AccelerationY]  "<AccelerationY>"
  Bus Selector/13 -> [AccelerationZ]  "<AccelerationZ>"
  Bus Selector/14 -> [WeightOnWheels]  "<WeightOnWheels>"
  Bus Selector/5 -> [FigureofMerit]  "<FigureofMerit>"
  Bus Selector1/1 -> [TRN_Ver_FlightPath_Angle]  "<TRN_Ver_FlightPath_Angle>"
  Bus Selector1/2 -> [TRNEstOfINSLatitudeErr]  "<TRNEstOfINSLatitudeErr>"
  Bus Selector1/3 -> [TRNEstOfINSLongitudeErr]  "<TRNEstOfINSLongitudeErr>"
  Bus Selector1/4 -> [TRNEstOfINSAltitudeErr]  "<TRNEstOfINSAltitudeErr>"
  Bus Selector1/5 -> [TRN_VelocityX]  "<TRN_VelocityX>"
  Bus Selector1/6 -> [TRN_VelocityY]  "<TRN_VelocityY>"
  Bus Selector1/7 -> [TRN_VelocityZ]  "<TRN_VelocityZ>"
  Bus Selector1/8 -> [TRNHorUncertainty]  "<TRNHorUncertainty>"
  Bus Selector1/9 -> [TRNVerticalUncertainty]  "<TRNVerticalUncertainty>"
  Bus Selector1/10 -> [TRN_Roll]  "<TRN_Roll>"
  Bus Selector1/11 -> [TRN_Pitch]  "<TRN_Pitch>"
  Bus Selector1/12 -> [TRN_Yaw]  "<TRN_Yaw>"
  Bus Selector1/13 -> [TRNEstOfLatitude]  "<TRNEstOfLatitude>"
  Bus Selector1/14 -> [TRNEstOfLongitude]  "<TRNEstOfLongitude>"
  Bus Selector1/15 -> [TRNEstHeightAGL]  "<TRNEstHeightAGL>"
  Bus Selector1/16 -> [NavigationMode]  "<NavigationMode>"
  Bus Selector1/17 -> [AircraftPositionCorrectionValid]  "<AircraftPositionCorrectionValid>"
  hDEM/1 -> [hDEM]
  Bus Selector/9 -> [RALTValid]  "<RALTValid>"
  [GPSDataNotValid] -> GPS/INS data + Acq CSU + Flag/1
  [P_code] -> GPS/INS data + Acq CSU + Flag/2
  [C_code] -> GPS/INS data + Acq CSU + Flag/3
  [FigureofMerit] -> GPS/INS data + Acq CSU + Flag/4
  [INSDataNotValid] -> GPS/INS data + Acq CSU + Flag/5
  [NavigationMode] -> GPS/INS data + Acq CSU + Flag/6
  [MAD] -> GPS/INS data + Acq CSU + Flag/8
  [profileCnt] -> GPS/INS data + Acq CSU + Flag/7
  [AircraftPositionCorrectionValid] -> GPS/INS data + Acq CSU + Flag/10
  [RALTValid] -> GPS/INS data + Acq CSU + Flag/11
  [WeightOnWheels] -> GPS/INS data + Acq CSU + Flag/12
  [TRNEstOfINSLatitudeErr] -> Subsystem7/1(In1)
  [TRNEstOfINSLongitudeErr] -> Subsystem7/2(In2)
  [TRNEstOfINSAltitudeErr] -> Subsystem7/3(In3)
  [Ref_lat] -> Subsystem7/4(4)
  [Ref_lon] -> Subsystem7/5(5)
  [Ref_alt] -> Subsystem7/6(6)
  [Latitude_INS] -> Subsystem7/7(7)
  [Longitude_INS] -> Subsystem7/8(8)
  [Altitude_INS] -> Subsystem7/9(9)
  [Latitude_GPS] -> Subsystem7/10(Lat_GPS)
  [Longitude_GPS] -> Subsystem7/11(Lon_GPS)
  [Altitude_GPS] -> Subsystem7/12(Alt_GPS)
  [TRNEstOfLatitude] -> Subsystem7/13(In13)
  [TRNEstOfLongitude] -> Subsystem7/14(In14)
  [TRN_MSL] -> Subsystem7/15(In15)
  [RALTAltitude] -> Subsystem7/16(RALT_AGL)
  [TRNEstHeightAGL] -> Subsystem7/17(TRN_AGL)
  Subsystem7/1(TRNCorr_INSErr_lat) -> TRN_Corr+INS_Err/1
  Subsystem7/2(TRNCorr_INSErr_lon) -> TRN_Corr+INS_Err/2
  Subsystem7/3(TRNCorr_INSErr_alt) -> TRN_Corr+INS_Err/3
  Subsystem7/4(Latitude) -> LLA/1
  Subsystem7/5(Longitude) -> LLA/2
  Subsystem7/6(Altitude) -> LLA/3
  Subsystem7/7(Comparison_AGL) -> LLA/4
  [hDEM] -> TRN Position error/4
  [TRNEstOfLatitude] -> Subsystem/1(In1)
  [Ref_lat] -> Subsystem/2(In2)
  [TRNEstOfLongitude] -> Subsystem/3(In3)
  [Ref_lon] -> Subsystem/4(In4)
  [TRN_MSL] -> Subsystem/5(In5)
  [Ref_alt] -> Subsystem/6(In6)
  Subsystem/1(TRN Position Error Horizon) -> TRN Position error/1
  Subsystem/2(TRN Position Error Vertical) -> TRN Position error/2
  Subsystem/3(Roughness) -> TRN Position error/3
  [Ref_roll] -> Subsystem2/1(1)
  [TRN_Roll] -> Subsystem2/2(2)
  [Ref_pitch] -> Subsystem2/3(3)
  [TRN_Pitch] -> Subsystem2/4(4)
  [Ref_yaw] -> Subsystem2/5(5)
  [TRN_Yaw] -> Subsystem2/6(6)
  [Ref_velX] -> Subsystem2/7(7)
  [TRN_VelocityX] -> Subsystem2/8(8)
  [Ref_velY] -> Subsystem2/9(9)
  [TRN_VelocityY] -> Subsystem2/10(10)
  [Ref_velZ] -> Subsystem2/11(11)
  [TRN_VelocityZ] -> Subsystem2/12(12)
  [Ref_accX] -> Subsystem2/13(13)
  [AccelerationX] -> Subsystem2/14(14)
  [Ref_accY] -> Subsystem2/15(15)
  [AccelerationY] -> Subsystem2/16(16)
  [Ref_accZ] -> Subsystem2/17(17)
  [AccelerationZ] -> Subsystem2/18(18)
  Subsystem2/1(Roll) -> Attitude + Velocity + Acceleration/1
  Subsystem2/2(Pitch) -> Attitude + Velocity + Acceleration/2
  Subsystem2/3(Yaw) -> Attitude + Velocity + Acceleration/3
  Subsystem2/4(Velocity X) -> Attitude + Velocity + Acceleration/4
  Subsystem2/5(Velocity Y) -> Attitude + Velocity + Acceleration/5
  Subsystem2/6(Velocity Z) -> Attitude + Velocity + Acceleration/6
  Subsystem2/7(Acceleration X) -> Attitude + Velocity + Acceleration/7
  Subsystem2/8(Acceleration Y) -> Attitude + Velocity + Acceleration/8
  Subsystem2/9(Acceleration Z) -> Attitude + Velocity + Acceleration/9
  [TimeTag_Prev] -> Terminator/1
  [TRN_Ver_FlightPath_Angle] -> Terminator2/1
  [TRNHorUncertainty] -> TRN Uncertainty/1
  [TRNVerticalUncertainty] -> TRN Uncertainty/2
  Bus Selector/15 -> [Latitude_INS]  "<Latitude_INS>"
  Bus Selector/16 -> [Longitude_INS]  "<Longitude_INS>"
  Bus Selector/17 -> [Altitude_INS]  "<Altitude_INS>"
  Bus Selector1/18 -> [TRN_valid]  "<TRN_valid>"
  [TRNOperatingEnv_Flag] -> GPS/INS data + Acq CSU + Flag/9
  [TRN_Roll] -> MATLAB Function/2(roll)
  [TRN_valid] -> MATLAB Function/1(TRN_valid)
  [INSDataNotValid] -> MATLAB Function/4(INSDataNotvalid)
  [TRN_Pitch] -> MATLAB Function/3(pitch)
  MATLAB Function/1(TRNOperatingEnv_Flag) -> [TRNOperatingEnv_Flag]
  [residual] -> Terminator1/1
  [TRN_VelocityZ] -> Subsystem5/12(12)
  [Latitude_GPS] -> Subsystem4/10(Lat_GPS)
  [Ref_pitch] -> Subsystem5/3(3)
  [Altitude_INS] -> Subsystem4/9(9)
  [Ref_yaw] -> Subsystem5/5(5)
  [Ref_alt] -> Subsystem4/6(6)
  [TRNEstOfINSLatitudeErr] -> Subsystem4/1(In1)
  [Ref_velY] -> Subsystem5/9(9)
  [TRNEstOfLatitude] -> Subsystem3/1(In1)
  [Latitude_INS] -> Subsystem4/7(7)
  [Longitude_GPS] -> Subsystem4/11(Lon_GPS)
  [Ref_roll] -> Subsystem5/1(1)
  [Ref_lat] -> Subsystem4/4(4)
  Subsystem3/3(Roughness) -> Bus Creator/3  "Roughness"
  [Ref_lon] -> Subsystem4/5(5)
  [TRN_MSL] -> Subsystem4/15(In15)
  [AccelerationX] -> Subsystem5/14(14)
  [Ref_velX] -> Subsystem5/7(7)
  [TRN_MSL] -> Subsystem3/5(In5)
  [TRN_VelocityX] -> Subsystem5/8(8)
  [Ref_accZ] -> Subsystem5/17(17)
  [RALTAltitude] -> Subsystem4/16(In16)
  [Ref_lat] -> Subsystem3/2(In2)
  [TRNEstOfINSAltitudeErr] -> Subsystem4/3(In3)
  [Altitude_GPS] -> Subsystem4/12(Alt_GPS)
  [INSDataNotValid] -> Bus Creator1/5
  [TRNEstOfLatitude] -> Subsystem4/13(In13)
  [NavigationMode] -> Bus Creator1/6
  [FigureofMerit] -> Bus Creator1/4
  [Ref_lon] -> Subsystem3/4(In4)
  [GPSDataNotValid] -> Bus Creator1/1
  [hDEM] -> Bus Creator/4
  [Ref_alt] -> Subsystem3/6(In6)
  [C_code] -> Bus Creator1/3
  [profileCnt] -> Bus Creator1/7
  [TRNEstOfLongitude] -> Subsystem4/14(In14)
  [Ref_accY] -> Subsystem5/15(15)
  [TRN_Yaw] -> Subsystem5/6(6)
  Subsystem3/2(TRN Position Error Vertical) -> Bus Creator/2  "TRNPositionError_Vertical"
  [Longitude_INS] -> Subsystem4/8(8)
  [RALTValid] -> Bus Creator1/11
  [TRNEstOfINSLongitudeErr] -> Subsystem4/2(In2)
  Subsystem5/9(Acceleration Z) -> Bus Creator4/9
  [Ref_accX] -> Subsystem5/13(13)
  [WeightOnWheels] -> Bus Creator1/12
  [P_code] -> Bus Creator1/2
  [MAD] -> Bus Creator1/8
  [TRN_VelocityY] -> Subsystem5/10(10)
  [TRNEstHeightAGL] -> Subsystem4/17(In17)
  Subsystem5/7(Acceleration X) -> Bus Creator4/7
  [TRN_Roll] -> Subsystem5/2(2)
  [AccelerationZ] -> Subsystem5/18(18)
  Subsystem5/4(Velocity X) -> Bus Creator4/4
  [AccelerationY] -> Subsystem5/16(16)
  Subsystem5/6(Velocity Z) -> Bus Creator4/6
  [TRNOperatingEnv_Flag] -> Bus Creator1/9
  [TRNEstOfLongitude] -> Subsystem3/3(In3)
  Subsystem5/2(Pitch) -> Bus Creator4/2
  Subsystem3/1(TRN Position Error Horizon) -> Bus Creator/1  "TRNPositionError_Horizon"
  [TRNVerticalUncertainty] -> Bus Creator3/2
  Subsystem5/5(Velocity Y) -> Bus Creator4/5
  Subsystem5/1(Roll) -> Bus Creator4/1
  [AircraftPositionCorrectionValid] -> Bus Creator1/10
  Subsystem5/3(Yaw) -> Bus Creator4/3
  [TRN_Pitch] -> Subsystem5/4(4)
  [Ref_velZ] -> Subsystem5/11(11)
  [TRNHorUncertainty] -> Bus Creator3/1
  Bus Creator/1 -> Bus Creator9/1  "TRNPosition_error"
  Bus Creator1/1 -> Bus Creator9/2  "GPS_INSData_AcqCSU_Flag"
  Bus Creator3/1 -> Bus Creator9/3  "TRNUncertainty"
  Subsystem5/8(Acceleration Y) -> Bus Creator4/8
  Bus Creator4/1 -> Bus Creator9/4  "Attitude_Velocity_Acceleration"
  Bus Creator9/1 -> To File/1
  Bus Selector/1 -> [INSDataNotValid]  "<INSDataNotValid>"
  Subsystem4/1(TRNCorr_INSErr_lat) -> Bus Creator5/1
  Subsystem4/2(TRNCorr_INSErr_lon) -> Bus Creator5/2
  Subsystem4/3(TRNCorr_INSErr_alt) -> Bus Creator5/3
  Bus Creator5/1 -> Bus Creator9/5  "TRNCorr_INSErr"
  Subsystem4/4(Latitude) -> Bus Creator6/1
  Subsystem4/5(Longitude) -> Bus Creator6/2
  Subsystem4/7(RALT_TRN_True_AGL) -> Bus Creator6/4
  Bus Creator6/1 -> Bus Creator9/6  "LLA"
  [TRN_IN] -> Subsystem4/18(TRN_IN)
  Subsystem7/8(RefGPS_Lat) -> Ref-GPS_LLA/1
  Subsystem7/9(RefGPS_Lon) -> Ref-GPS_LLA/2
  Subsystem7/10(RefGPS_Alt) -> Ref-GPS_LLA/3
  Subsystem4/8(INSGPS_Err) -> Bus Creator7/1  "INSGPS_Err"
  Subsystem4/6(Altitude) -> Bus Creator6/3
  Bus Creator7/1 -> Bus Creator9/7  "INSGPS_Err"
  Subsystem4/9(GPSEstUncer) -> Bus Creator7/2  "GPSEstUncer"
  [hDEM] -> Subsystem7/18(hDEM)
  Subsystem7/11(out_hDEM) -> Altitude Comparison/1
  [Altitude_INS] -> Altitude Comparison/2
  [TRN_MSL] -> Altitude Comparison/3
  Subsystem7/12(hDEM+RALT) -> Altitude Comparison/4
  [Ref_alt] -> Altitude Comparison/5
  [hDEM] -> Subsystem4/19(hDEM)
  Subsystem4/10(out_hDEM) -> Bus Creator8/1  "Ref_hDEM"
  [Altitude_INS] -> Bus Creator8/2  "Altitude_INS"
  [TRN_MSL] -> Bus Creator8/3  "TRN_MSL"
  [Ref_alt] -> Bus Creator8/5  "Ref_Alt"
  Subsystem4/11(hDEM+RALT) -> Bus Creator8/4  "RALT_hDEM"
  Bus Creator8/1 -> Bus Creator9/8  "Altitude_Comparison"

== system TRN_KAISIM/TRN/Terrain_Func ==
  lat : Inport
  lon : Inport  Port=2
  CheckOffTerrainMap : MATLAB Function  TreatAsAtomicUnit=on
      settings: RTWSystemCode=Nonreusable function  RTWFcnNameOpts=Use subsystem name
  FTGMapCaching : MATLAB Function  TreatAsAtomicUnit=on
  Scope : Scope  NumInputPorts=2
  Terminator : Terminator
  Terminator1 : Terminator
  Terrain_Level_big : MATLAB Function  TreatAsAtomicUnit=on
  updateFlag : MATLAB Function  TreatAsAtomicUnit=on
      settings: RTWSystemCode=Nonreusable function  RTWFcnNameOpts=Use subsystem name
  hdem : Outport
  Updateflag : Outport  Port=2
  AircraftOffTerrainMap : Outport  Port=3
  wires:
  lat/1 -> Terrain_Level_big/1(Lat), FTGMapCaching/1(lat)
  FTGMapCaching/3(hDEM) -> Scope/1, CheckOffTerrainMap/1(hDEM), hdem/1
  lon/1 -> Terrain_Level_big/2(Lon), FTGMapCaching/2(lon)
  Terrain_Level_big/1(R) -> Scope/2, updateFlag/2(roughness)
  FTGMapCaching/1(resultDTED) -> Terminator/1
  FTGMapCaching/2(resultDVOF) -> Terminator1/1
  CheckOffTerrainMap/1(AircraftOffTerrainMap) -> updateFlag/1(AircraftOffTerrainMap), AircraftOffTerrainMap/1
  updateFlag/1(UpdateFlag) -> Updateflag/1

== system TRN_KAISIM/TRN/ModeManagementCSU/AcquisitionCSU/AcquisitionCSU ==
  In_TRNInput : Inport  OutDataTypeStr=Bus: TRNInput
  In_TRNDatapump : Inport  Port=2  OutDataTypeStr=Bus: TRNDatapump
  Bus Selector2 : BusSelector  OutputSignals=profileCnt,Result_Prev
  CollectProfile : MATLAB Function  TreatAsAtomicUnit=on
      settings: RTWSystemCode=Nonreusable function  RTWFcnNameOpts=Use subsystem name
  ConvertTRNInput : Subsystem  TreatAsAtomicUnit=on
  CorrelationAnalysis : MATLAB Function  TreatAsAtomicUnit=on
      settings: RTWSystemCode=Nonreusable function  RTWFcnNameOpts=Use subsystem name
  Data Store Read : DataStoreRead  DataStoreName=BatchProf  IndexOptions=Index vector (dialog)  Indices=1  OutputSizes=1
  Data Store Read1 : DataStoreRead  DataStoreName=profileLimit  IndexOptions=Index vector (dialog)  Indices=1  OutputSizes=1
  Data Store Read10 : DataStoreRead  DataStoreName=gridRes  IndexOptions=Index vector (dialog)  Indices=1  OutputSizes=1
  Data Store Read11 : DataStoreRead  DataStoreName=gridSize  IndexOptions=Index vector (dialog)  Indices=1  OutputSizes=1
  Data Store Read3 : DataStoreRead  DataStoreName=gridSize  IndexOptions=Index vector (dialog)  Indices=1  OutputSizes=1
  Data Store Read4 : DataStoreRead  DataStoreName=gridRes  IndexOptions=Index vector (dialog)  Indices=1  OutputSizes=1
  Data Store Read5 : DataStoreRead  DataStoreName=RES  IndexOptions=Index vector (dialog)  Indices=1  OutputSizes=1
  Data Store Read9 : DataStoreRead  DataStoreName=RES  IndexOptions=Index vector (dialog)  Indices=1  OutputSizes=1
  Data Store Write : DataStoreWrite  DataStoreName=BatchProf  IndexOptions=Index vector (dialog)  Indices=1  OutputSizes=1
  Data Type Conversion : DataTypeConversion  OutDataTypeStr=boolean  SaturateOnIntegerOverflow=off  RndMeth=Floor
  Demux : Demux  Outputs=6
  MAPValid : MATLAB Function  TreatAsAtomicUnit=on
  Mux : Mux
  NOT : Logic  Operator=NOT  IconShape=distinctive  AllPortsSameDT=off  OutDataTypeStr=boolean
  SetProfile : MATLAB Function  TreatAsAtomicUnit=on
      settings: RTWSystemCode=Nonreusable function  RTWFcnNameOpts=Use subsystem name
  StoreProfile : MATLAB Function  TreatAsAtomicUnit=on
      settings: RTWSystemCode=Nonreusable function  RTWFcnNameOpts=Use subsystem name
  Terminator3 : Terminator
  Terminator4 : Terminator
  MAD : Outport  VectorParamsAs1DForOutWhenUnconnected=off
  profileCnt : Outport  Port=2  VectorParamsAs1DForOutWhenUnconnected=off
  posUpdate : Outport  Port=3  VectorParamsAs1DForOutWhenUnconnected=off
  residual : Outport  Port=4  VectorParamsAs1DForOutWhenUnconnected=off
  wires:
  Data Store Read5/1 -> CollectProfile/4(resolution)
  Data Store Read4/1 -> CollectProfile/5(gridRes)
  Data Store Read9/1 -> CorrelationAnalysis/4(resolution)
  Data Store Read10/1 -> CorrelationAnalysis/5(gridRes)
  Data Store Read11/1 -> CorrelationAnalysis/3(gridSize)
  CollectProfile/2(batchProfile) -> Data Store Write/1, CorrelationAnalysis/1(batchProfile)
  CorrelationAnalysis/1(posUpdate) -> posUpdate/1
  CorrelationAnalysis/2(MAD) -> MAD/1
  CorrelationAnalysis/3(residual) -> residual/1
  Data Store Read/1 -> SetProfile/1("batchProfile ")
  Bus Selector2/1 -> SetProfile/2("profileCnt ")  "<profileCnt>"
  ConvertTRNInput/4(altRALT) -> StoreProfile/5(RALT)
  In_TRNInput/1 -> ConvertTRNInput/1(TRNInput)
  In_TRNDatapump/1 -> Bus Selector2/1
  SetProfile/1(batchProfile) -> StoreProfile/12("batchProfile ")
  SetProfile/2(profileCnt) -> StoreProfile/13("profileCnt ")
  ConvertTRNInput/1(latINS) -> StoreProfile/2(latINS)
  ConvertTRNInput/2(lonINS) -> StoreProfile/3(lonINS)
  ConvertTRNInput/3(altINS) -> StoreProfile/4(altINS)
  ConvertTRNInput/5(latGPS) -> StoreProfile/6(latGPS)
  ConvertTRNInput/6(lonGPS) -> StoreProfile/7(lonGPS)
  ConvertTRNInput/7(altGPS) -> StoreProfile/8(altGPS)
  ConvertTRNInput/8(GPSDataNotValid) -> StoreProfile/9(GPSDataNotValid)
  ConvertTRNInput/9(INSDataNotValid) -> StoreProfile/10(INSDataNotValid)
  StoreProfile/1(profileCnt) -> CorrelationAnalysis/2(profileCnt), profileCnt/1, CollectProfile/1(profileCnt)
  StoreProfile/3(gridSize) -> CollectProfile/3(gridSize)
  StoreProfile/2(batchProfile) -> CollectProfile/2("batchProfile ")
  ConvertTRNInput/10(FigureofMerit) -> StoreProfile/11(GPSFoM)
  Demux/1 -> Data Type Conversion/1
  Bus Selector2/2 -> Demux/1  "<Result_Prev>"
  Mux/1 -> Terminator3/1
  Data Type Conversion/1 -> MAPValid/1(In_MAPValid)
  MAPValid/1(MAPValid) -> StoreProfile/15(MAPvalidFlag)
  Data Store Read3/1 -> SetProfile/3("gridSize ")
  SetProfile/3(gridSize) -> StoreProfile/14("gridSize ")
  Data Store Read1/1 -> SetProfile/4(profileLimit)
  NOT/1 -> StoreProfile/1(firstRun)
  Demux/2 -> NOT/1
  Demux/3 -> Mux/1
  Demux/4 -> Mux/2
  Demux/5 -> Mux/3
  Demux/6 -> Mux/4
  CollectProfile/1(hDEM) -> Terminator4/1
